simulink model "BME 306_project_1818027"  (R2022b)
settings: Solver=VariableStepAuto  StartTime=0.0  StopTime=10.0  RelTol=1e-3
libraries: simulink x1
settings Model: Creator=HP  LastModifiedBy=HP

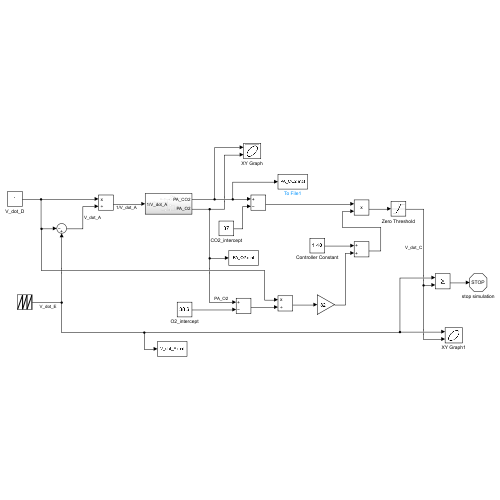
[thumbnail: Simulink's stored preview of the top-level diagram]
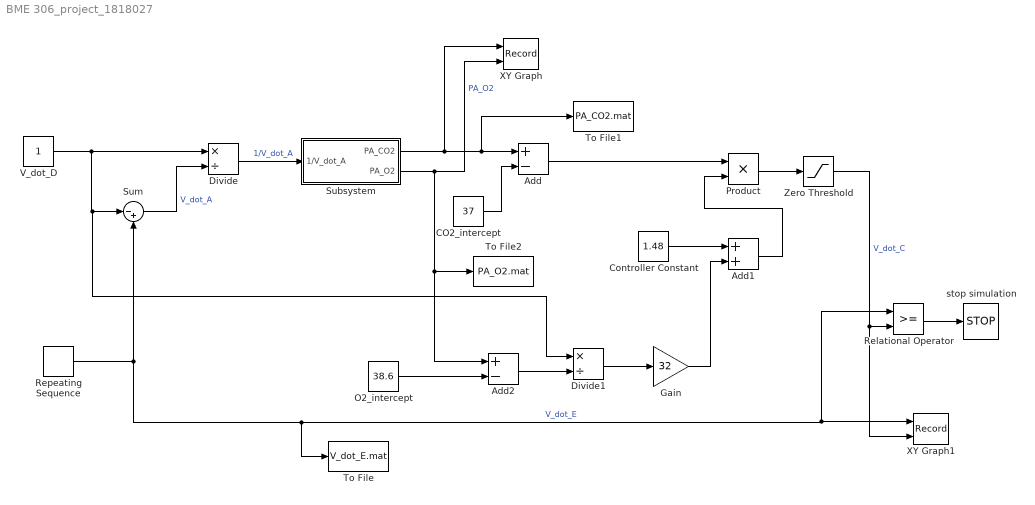
== system BME 306_project_1818027 ==
  Add : Sum  Inputs=+-
  Add1 : Sum
  Add2 : Sum  Inputs=+-
  CO2_intercept : Constant  Value=37
  Controller Constant : Constant  Value=1.48
  Divide : Product  Inputs=*/
  Divide1 : Product  Inputs=*/
  Gain : Gain  Gain=32
  O2_intercept : Constant  Value=38.6
  Product : Product
  Relational Operator : RelationalOperator  OutDataTypeStr=boolean  RndMeth=Simplest  InputSameDT=off
  Repeating Sequence : simulink/Sources/Repeating Sequence  rep_seq_t=[0 10]  rep_seq_y=[4 10]
  Subsystem : Subsystem
  Sum : Sum  Inputs=|-+
  To File : ToFile  Filename=V_dot_E.mat  SaveFormat=Timeseries
  To File1 : ToFile  Filename=PA_CO2.mat  SaveFormat=Timeseries
  To File2 : ToFile  Filename=PA_O2.mat  SaveFormat=Timeseries
  V_dot_D : Constant
  XY Graph : Record  FileSettingsInternal="{\"entries\":[{\"content\":{\"excelSettings\":{\"content\":{},\"type\":\"Streamout.ExcelSettings\"}},\"type\":\"Streamout.FileSettingStorage\",\"uuid\":\"81a3149f-6ff3-4546-b31e-e467cdc3dbb0\"}],\"packageUris\":[\"http://schema.mathworks.com/mf0/streamout_blocks/R2020a\"],\"version\":\"1.0\"}"  Layout=[1 1]  SignalsInternal="{\"entries\":[{\"content\":{\"signals\":[{\"content\":{\"blockPath\":[\"project_1818027/XY Graph\"],\"channel\":[],\"dimensions\":[1],\"domain\":\"project_1818027/XY Graph\",\"lineColor\":\"#a2142f\",\"plots\":[1],\"port\":1,\"sid\":[\"\"],\"signalID\":68,\"signalName\":\"Subsystem:1\"},\"type\":\"RecordBlkView.Signal\",\"uuid\":\"84af3b74-4cac-4756-9d36-38824816c752\"},{\"content\":{\"blockPath\":[\"project_1818027/XY Graph\"],\"channel\":[],\"dimensions\":[1],\"domain\":\"project_1818027/XY Graph\",\"lineColor\":\"#139fff\",\"plots\":[1],\"port\":2,\"sid\":[\"\"],\"signalID\":72,\"signalName\":\"PA_O2\"},\"type\":\"RecordBlkView.Signal\",\"uuid\":\"1c98abfd-7662-4300-bfa8-8729cc1c5726\"}]},\"type\":\"RecordBlkView.InputSignals\",\"uuid\":\"6278fb0d-b897-46db-9c74-da83c9b7a3c4\"}],\"packageUris\":[\"http://schema.mathworks.com/mf0/streamout_blocks/R2020a\"],\"version\":\"1.0\"}"  VisualizationBindings="{\"xyplotplugin\":{\"info\":[{\"series\":[{\"bindingParametersList\":[{\"parameter\":\"X-Axis\",\"signalID\":68,\"signalName\":\"Subsystem:1\"},{\"parameter\":\"Y-Axis\",\"signalID\":72,\"signalName\":\"PA_O2\"}],\"seriesID\":20253}],\"subplotID\":1}]}}"  CompatibilityTag=XY
  XY Graph1 : Record  FileSettingsInternal="{\"entries\":[{\"content\":{\"excelSettings\":{\"content\":{},\"type\":\"Streamout.ExcelSettings\"}},\"type\":\"Streamout.FileSettingStorage\",\"uuid\":\"b4c82504-c5ee-476a-86e2-babfc9d21630\"}],\"packageUris\":[\"http://schema.mathworks.com/mf0/streamout_blocks/R2020a\"],\"version\":\"1.0\"}"  Layout=[1 1]  SignalsInternal="{\"entries\":[{\"content\":{\"signals\":[{\"content\":{\"blockPath\":[\"project_1818027/XY Graph1\"],\"channel\":[],\"dimensions\":[1],\"domain\":\"project_1818027/XY Graph1\",\"lineColor\":\"#a2142f\",\"plots\":[1],\"port\":1,\"sid\":[\"\"],\"signalID\":76,\"signalName\":\"V_dot_E\"},\"type\":\"RecordBlkView.Signal\",\"uuid\":\"d94f61b9-f15c-4244-98d6-26cdee56de4c\"},{\"content\":{\"blockPath\":[\"project_1818027/XY Graph1\"],\"channel\":[],\"dimensions\":[1],\"domain\":\"project_1818027/XY Graph1\",\"lineColor\":\"#139fff\",\"plots\":[1],\"port\":2,\"sid\":[\"\"],\"signalID\":80,\"signalName\":\"V_dot_C\"},\"type\":\"RecordBlkView.Signal\",\"uuid\":\"ad3d07c3-cb3a-403f-9901-59e210bb7ddc\"}]},\"type\":\"RecordBlkView.InputSignals\",\"uuid\":\"66dd1afc-3210-4bab-8198-1a090809ccda\"}],\"packageUris\":[\"http://schema.mathworks.com/mf0/streamout_blocks/R2020a\"],\"version\":\"1.0\"}"  VisualizationBindings="{\"xyplotplugin\":{\"info\":[{\"series\":[{\"bindingParametersList\":[{\"parameter\":\"X-Axis\",\"signalID\":76,\"signalName\":\"V_dot_E\"},{\"parameter\":\"Y-Axis\",\"signalID\":80,\"signalName\":\"V_dot_C\"}],\"seriesID\":64281}],\"subplotID\":1}]}}"  CompatibilityTag=XY
  Zero Threshold : Saturate  UpperLimit=20  LowerLimit=0
  stop simulation : Stop
  wires:
  Repeating Sequence/1 -> Sum/2, To File/1, XY Graph1/1, Relational Operator/1  "V_dot_E"
  Sum/1 -> Divide/2  "V_dot_A"
  Divide/1 -> Subsystem/1(1/V_dot_A)  "1/V_dot_A"
  Subsystem/1(PA_CO2) -> XY Graph/1, To File1/1, Add/1
  Subsystem/2(PA_O2) -> XY Graph/2, To File2/1, Add2/1  "PA_O2"
  CO2_intercept/1 -> Add/2
  Controller Constant/1 -> Add1/1
  Add1/1 -> Product/2
  Add/1 -> Product/1
  O2_intercept/1 -> Add2/2
  Add2/1 -> Divide1/2
  Divide1/1 -> Gain/1
  Gain/1 -> Add1/2
  Product/1 -> Zero Threshold/1
  Zero Threshold/1 -> XY Graph1/2, Relational Operator/2  "V_dot_C"
  Relational Operator/1 -> stop simulation/1
  V_dot_D/1 -> Divide/1, Divide1/1, Sum/1

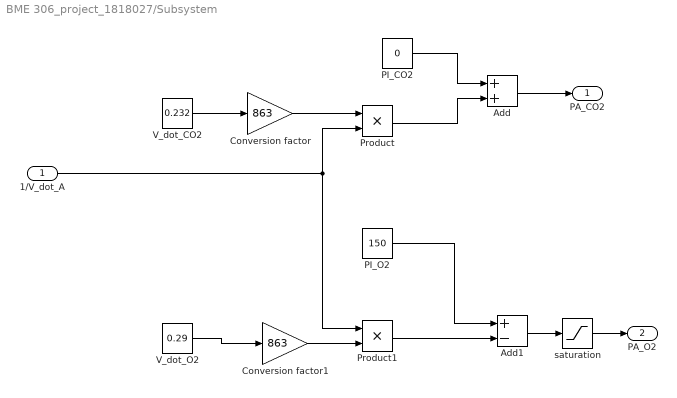
== system BME 306_project_1818027/Subsystem ==
  1/V_dot_A : Inport
  Add : Sum
  Add1 : Sum  Inputs=+-
  Conversion factor : Gain  Gain=863
  Conversion factor1 : Gain  Gain=863
  PI_CO2 : Constant  Value=0
  PI_O2 : Constant  Value=150
  Product : Product
  Product1 : Product
  V_dot_CO2 : Constant  Value=0.232
  V_dot_O2 : Constant  Value=0.29
  saturation : Saturate  UpperLimit=150  LowerLimit=40
  PA_CO2 : Outport
  PA_O2 : Outport  Port=2
  wires:
  1/V_dot_A/1 -> Product/2, Product1/1
  Product/1 -> Add/2
  Product1/1 -> Add1/2
  Conversion factor/1 -> Product/1
  V_dot_O2/1 -> Conversion factor1/1
  Add1/1 -> saturation/1
  PI_CO2/1 -> Add/1
  PI_O2/1 -> Add1/1
  V_dot_CO2/1 -> Conversion factor/1
  Conversion factor1/1 -> Product1/2
  Add/1 -> PA_CO2/1
  saturation/1 -> PA_O2/1
